simulink model "thermostat_sf"  (Simulink 4.00)
settings: Solver=ode45  StartTime=0.0  StopTime=10.0  RelTol=1e-1
settings Model: LastModifiedBy=hespanha  LimitDataPoints=off  ExtModeTrigMode=oneshot  ExtModeArmWhenConnect=off  BlockReductionOpt=off

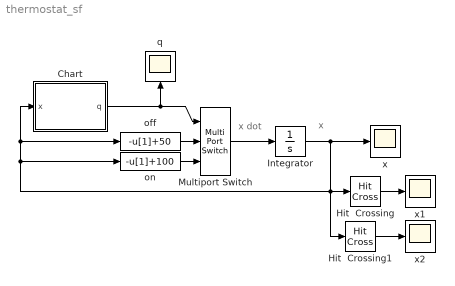
== system thermostat_sf ==
  note: x
  note: x dot
  Chart : Stateflow chart
      settings: RTWFcnNameOpts=Auto  RTWFileNameOpts=Auto
  Hit  Crossing : HitCross  HitCrossingOffset=77  HitCrossingDirection=rising  ShowOutputPort=on
  Hit  Crossing1 : HitCross  HitCrossingOffset=73  HitCrossingDirection=falling  ShowOutputPort=on
  Integrator : Integrator  ExternalReset=none  InitialConditionSource=internal  InitialCondition=0  LimitOutput=off  UpperSaturationLimit=inf  LowerSaturationLimit=-inf  ShowSaturationPort=off  ShowStatePort=off  AbsoluteTolerance=auto
  Multiport Switch : MultiPortSwitch  Inputs=2
  off : Fcn  Expr=-u[1]+50
  on : Fcn  Expr=-u[1]+100
  q : Scope
      settings: Orientation=up  TimeRange=10  YMin=0  YMax=3  SaveToWorkspace=off  SaveName=ScopeData  LimitDataPoints=on  MaxDataPoints=5000
  x : Scope
      settings: TimeRange=10  YMin=0  YMax=80  SaveToWorkspace=off  SaveName=ScopeData  LimitDataPoints=on  MaxDataPoints=5000
  x1 : Scope
      settings: TimeRange=10  YMin=-1  YMax=2  SaveToWorkspace=off  LimitDataPoints=on  MaxDataPoints=5000
  x2 : Scope
      settings: TimeRange=10  YMin=-1  YMax=2  SaveToWorkspace=off  SaveName=ScopeData2  LimitDataPoints=on  MaxDataPoints=5000
  wires:
  Multiport Switch/1 -> Integrator/1
  Chart/1(q) -> Multiport Switch/1, q/1
  off/1 -> Multiport Switch/2
  on/1 -> Multiport Switch/3
  Integrator/1 -> x/1, Chart/1(x), off/1, on/1, Hit  Crossing/1, Hit  Crossing1/1
  Hit  Crossing/1 -> x1/1
  Hit  Crossing1/1 -> x2/1

== stateflow chart Chart ==
  state off/
    entry:q=1;
  state on/
    entry:q=2;
  (default) -> off
  off -> on : [x<=73]
  on -> off : [x>=77]
  data: q output int8; x input double
